simulink model "IPC_fullIPC"  (R2022a)
settings: Solver=FixedStepDiscrete  StartTime=0.0  StopTime=TMax  FixedStep=DT  RelTol=1e-3
undefined symbols (not defined in the file): DiscIntNeverNeededParam, Ki, optimal_azimuth_offset_rad
settings Model: Creator=jhummel  LastModifiedBy=jhummel

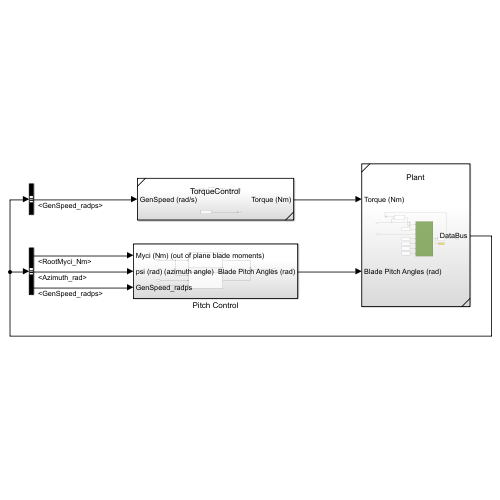
[thumbnail: Simulink's stored preview of the top-level diagram]
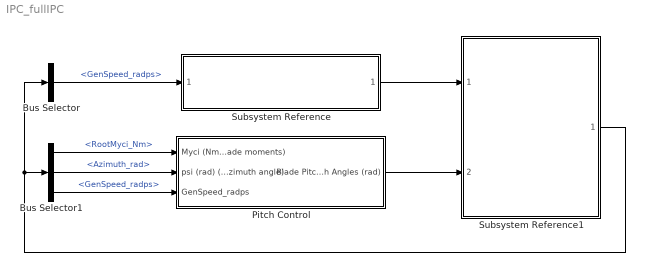
== system IPC_fullIPC ==
  Bus Selector : BusSelector  OutputSignals=GenSpeed_radps
  Bus Selector1 : BusSelector  OutputSignals=RootMyci_Nm,Azimuth_rad,GenSpeed_radps
  Pitch Control : Subsystem
  Subsystem Reference : Subsystem  ReferencedSubsystem=TorqueControl
  Subsystem Reference1 : Subsystem  ReferencedSubsystem=Plant
  wires:
  Bus Selector/1 -> Subsystem Reference/1  "<GenSpeed_radps>"
  Bus Selector1/1 -> Pitch Control/1(Myci (Nm) (out of plane blade moments))  "<RootMyci_Nm>"
  Bus Selector1/2 -> Pitch Control/2(psi (rad) (azimuth angle))  "<Azimuth_rad>"
  Bus Selector1/3 -> Pitch Control/3(GenSpeed_radps)  "<GenSpeed_radps>"
  Subsystem Reference1/1 -> Bus Selector/1, Bus Selector1/1
  Pitch Control/1(Blade Pitch Angles (rad)) -> Subsystem Reference1/2
  Subsystem Reference/1 -> Subsystem Reference1/1

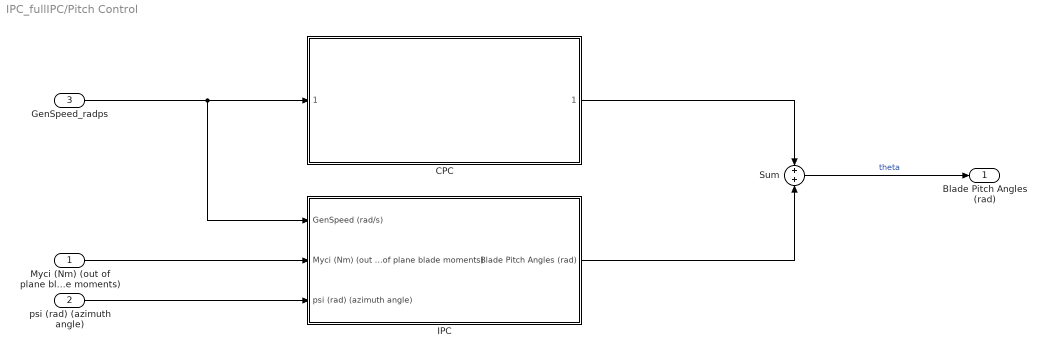
== system IPC_fullIPC/Pitch Control ==
  Myci (Nm) (out of plane blade moments) : Inport
  psi (rad) (azimuth angle) : Inport  Port=2
  GenSpeed_radps : Inport  Port=3
  CPC : Subsystem  ReferencedSubsystem=CollectivePitchControl
  IPC : Subsystem
  Sum : Sum  Inputs=+|+
  Blade Pitch Angles (rad) : Outport
  wires:
  Myci (Nm) (out of plane blade moments)/1 -> IPC/2(Myci (Nm) (out of plane blade moments))
  psi (rad) (azimuth angle)/1 -> IPC/3(psi (rad) (azimuth angle))
  GenSpeed_radps/1 -> IPC/1(GenSpeed (rad/s)), CPC/1
  IPC/1(Blade Pitch Angles (rad)) -> Sum/2
  Sum/1 -> Blade Pitch Angles (rad)/1  "theta"
  CPC/1 -> Sum/1

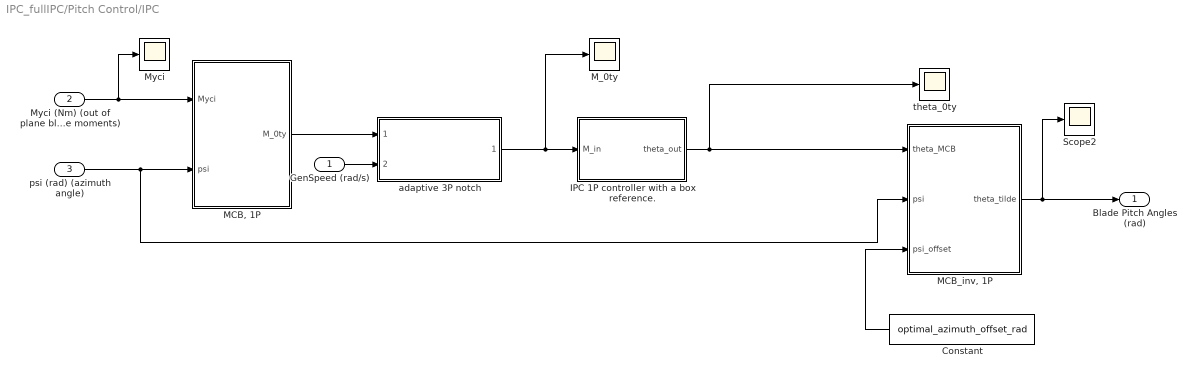
== system IPC_fullIPC/Pitch Control/IPC ==
  GenSpeed (rad/s) : Inport
  Myci (Nm) (out of plane blade moments) : Inport  Port=2
  psi (rad) (azimuth angle) : Inport  Port=3
  Constant : Constant  Value=optimal_azimuth_offset_rad
  IPC 1P controller with a box reference. : Subsystem
  "MCB, 1P" : MATLAB Function  TreatAsAtomicUnit=on
  "MCB_inv, 1P" : MATLAB Function  TreatAsAtomicUnit=on
  M_0ty : Scope
  Myci : Scope
  Scope2 : Scope
  adaptive 3P notch : Subsystem  ReferencedSubsystem=LoadFilter
  theta_0ty : Scope
  Blade Pitch Angles (rad) : Outport
  wires:
  Myci (Nm) (out of plane blade moments)/1 -> Myci/1, "MCB, 1P"/1(Myci)
  "MCB_inv, 1P"/1(theta_tilde) -> Blade Pitch Angles (rad)/1, Scope2/1
  "MCB, 1P"/1(M_0ty) -> adaptive 3P notch/1
  psi (rad) (azimuth angle)/1 -> "MCB_inv, 1P"/2(psi), "MCB, 1P"/2(psi)
  IPC 1P controller with a box reference./1(theta_out) -> "MCB_inv, 1P"/1(theta_MCB), theta_0ty/1
  adaptive 3P notch/1 -> M_0ty/1, IPC 1P controller with a box reference./1(M_in)
  GenSpeed (rad/s)/1 -> adaptive 3P notch/2
  Constant/1 -> "MCB_inv, 1P"/3(psi_offset)

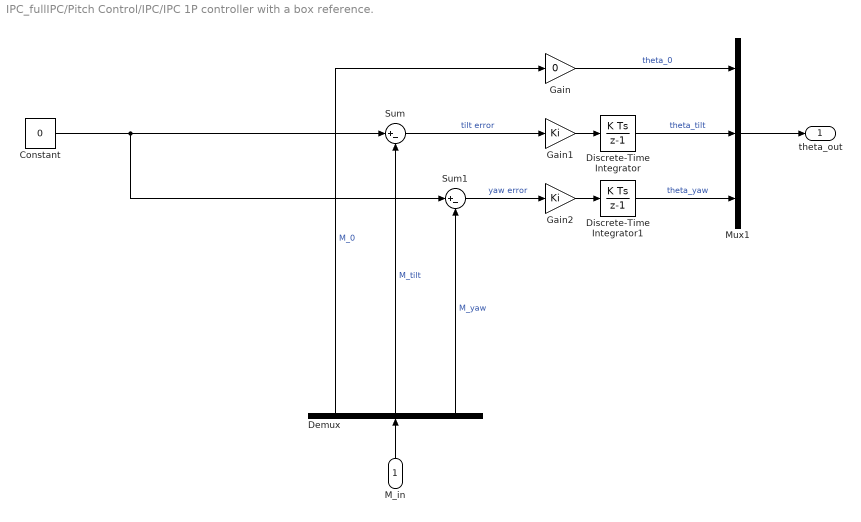
== system IPC_fullIPC/Pitch Control/IPC/IPC 1P controller with a box reference. ==
  M_in : Inport
  Constant : Constant  Value=0
  Demux : Demux  Outputs=3
  Discrete-Time Integrator : DiscreteIntegrator  SampleTime=-1  ICPrevOutput=DiscIntNeverNeededParam  ICPrevScaledInput=DiscIntNeverNeededParam
  Discrete-Time Integrator1 : DiscreteIntegrator  SampleTime=-1  ICPrevOutput=DiscIntNeverNeededParam  ICPrevScaledInput=DiscIntNeverNeededParam
  Gain : Gain  Gain=0
  Gain1 : Gain  Gain=Ki
  Gain2 : Gain  Gain=Ki
  Mux1 : Mux  Inputs=3
  Sum : Sum  Inputs=|+-
  Sum1 : Sum  Inputs=|+-
  theta_out : Outport
  wires:
  Gain/1 -> Mux1/1  "theta_0"
  Demux/1 -> Gain/1  "M_0"
  Demux/2 -> Sum/2  "M_tilt"
  Demux/3 -> Sum1/2  "M_yaw"
  Sum/1 -> Gain1/1  "tilt error"
  Sum1/1 -> Gain2/1  "yaw error"
  M_in/1 -> Demux/1
  Mux1/1 -> theta_out/1
  Discrete-Time Integrator/1 -> Mux1/2  "theta_tilt"
  Discrete-Time Integrator1/1 -> Mux1/3  "theta_yaw"
  Constant/1 -> Sum1/1, Sum/1
  Gain1/1 -> Discrete-Time Integrator/1
  Gain2/1 -> Discrete-Time Integrator1/1

== matlab function IPC_fullIPC/Pitch Control/IPC/MCB_inv, 1P ==
  data: theta_MCB input; psi input; psi_offset input; theta_tilde output
function theta_tilde = fcn(theta_MCB, psi, psi_offset)

theta_tilde = MBC_inv(theta_MCB, psi, psi_offset, 3, 1);

end

== matlab function IPC_fullIPC/Pitch Control/IPC/MCB, 1P ==
  data: Myci input; M_0ty output; psi input
function M_0ty = fcn(Myci, psi)

% Do the coordinate transformation.
M_0ty = MBC(Myci, psi, 0, 3, 1);

end
